simulink model "coffee_machine"  (R2024b)
settings: Solver=ode45  StartTime=0.0  StopTime=10.0  RelTol=1e-3
settings Model: Creator=HP  LastModifiedBy=HP

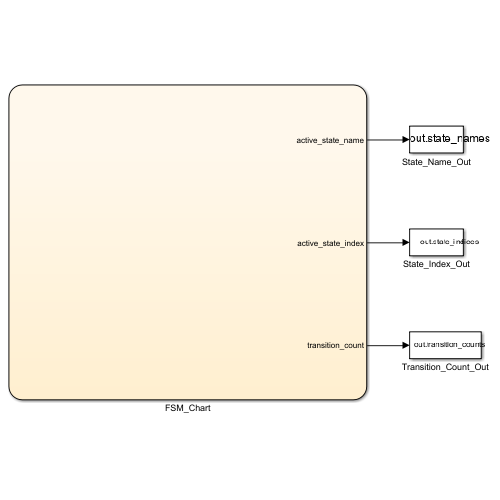
[thumbnail: Simulink's stored preview of the top-level diagram]
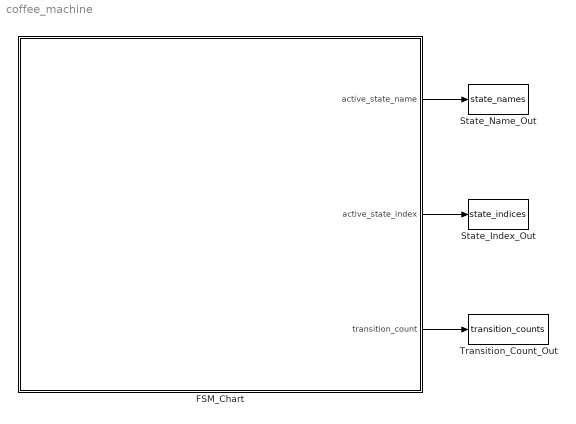
== system coffee_machine ==
  FSM_Chart : Stateflow chart  TreatAsAtomicUnit=on
  State_Index_Out : ToWorkspace  VariableName=state_indices  SaveFormat=Timeseries  SampleTime=-1
  State_Name_Out : ToWorkspace  VariableName=state_names  SaveFormat=Timeseries  SampleTime=-1
  Transition_Count_Out : ToWorkspace  VariableName=transition_counts  SaveFormat=Timeseries  SampleTime=-1
  wires:
  FSM_Chart/1(active_state_name) -> State_Name_Out/1
  FSM_Chart/2(active_state_index) -> State_Index_Out/1
  FSM_Chart/3(transition_count) -> Transition_Count_Out/1

== stateflow chart coffee_machine/FSM_Chart ==
  state entry_1 active_state_name = "MakingCoffee"; active_state_index = 2;\nentry: try; print(""Starting coffee making process...""); catch; end;\nexit: try; print(""Coffee process finished.""); credit = 0; catch; end;
    settings: description=A superstate that encapsulates the multi-step coffee making process.
    state entry_2 active_state_name = "Idle"; active_state_index = 3;\nentry: try; print(""Machine is Idle.""); credit = 0; catch; end;\nexit: try; print(""Leaving Idle state.""); catch; end;
      settings: description=The machine is waiting for a coin.
    state entry_ active_state_name = "HasCredit"; active_state_index = 1;\nentry: try; print(f""Credit is now: {credit}""); catch; end;
      settings: description=The machine has received payment and is waiting for a selection.
    entry_1 active_state_name = "MakingCoffee"; active_state_index = 2;\nentry: try; print(""Starting coffee making process...""); catch; end;\nexit: try; print(""Coffee process finished.""); credit = 0; catch; end; -> entry_2 active_state_name = "Idle"; active_state_index = 3;\nentry: try; print(""Machine is Idle.""); credit = 0; catch; end;\nexit: try; print(""Leaving Idle state.""); catch; end; : /{try; print(""Dispensing complete. Returning to Idle.""); catch; end; trans_count_local = trans_count_local + 1; transition_count = trans_count_local}
      settings: description=Transition from MakingCoffee to Idle
    entry_ active_state_name = "HasCredit"; active_state_index = 1;\nentry: try; print(f""Credit is now: {credit}""); catch; end; -> entry_2 active_state_name = "Idle"; active_state_index = 3;\nentry: try; print(""Machine is Idle.""); credit = 0; catch; end;\nexit: try; print(""Leaving Idle state.""); catch; end; [order 1] : cancel /{try; print(f""Returning {credit} credit(s).""); credit = 0; catch; end; trans_count_local = trans_count_local + 1; transition_count = trans_count_local}
      settings: description=Transition from HasCredit to Idle
    entry_2 active_state_name = "Idle"; active_state_index = 3;\nentry: try; print(""Machine is Idle.""); credit = 0; catch; end;\nexit: try; print(""Leaving Idle state.""); catch; end; -> entry_ active_state_name = "HasCredit"; active_state_index = 1;\nentry: try; print(f""Credit is now: {credit}""); catch; end; : insert_coin /{try; credit = credit + 1; catch; end; trans_count_local = trans_count_local + 1; transition_count = trans_count_local}
      settings: description=Transition from Idle to HasCredit
    entry_ active_state_name = "HasCredit"; active_state_index = 1;\nentry: try; print(f""Credit is now: {credit}""); catch; end; -> entry_1 active_state_name = "MakingCoffee"; active_state_index = 2;\nentry: try; print(""Starting coffee making process...""); catch; end;\nexit: try; print(""Coffee process finished.""); credit = 0; catch; end; [order 2] : select_coffee [credit >= 1] /{try; print(""Selection made with sufficient credit.""); catch; end; trans_count_local = trans_count_local + 1; transition_count = trans_count_local}
      settings: description=Transition from HasCredit to MakingCoffee
  (default) -> entry_2 active_state_name = "Idle"; active_state_index = 3;\nentry: try; print(""Machine is Idle.""); credit = 0; catch; end;\nexit: try; print(""Leaving Idle state.""); catch; end; : [trans_count_local = 0]
    settings: description=Initial transition to Idle
  data: active_state_name output string; active_state_index output uint8; transition_count output uint32; trans_count_local local uint32
